simulink model "frdm_main"  (R2017a)
settings: Solver=FixedStepAuto  StartTime=0.0  StopTime=inf  RelTol=1e-3  EnableMultiTasking=on
libraries: frdmtfcshieldlib x5, frdmkl25zlib x2
settings Model: SimulationMode=external  ExtModeTrigDuration=5  Creator=WARA  LastModifiedBy=WARA
settings OptimizationCC: PassReuseOutputArgsThreshold=0  MaxStackSize=64
settings DebuggingCC: ParameterTunabilityLossMsg=error
settings HardwareCC: ProdBitPerPointer=32  ProdBitPerSizeT=32  ProdBitPerPtrDiffT=32  ProdLargestAtomicInteger=Long  ProdLargestAtomicFloat=Double  ProdWordSize=32  ProdHWDeviceType=ARM Compatible->ARM Cortex  UseEmbeddedCoderFeatures=off
settings SFSimCC: MATLABDynamicMemAlloc=off
settings RTWCC: SystemTargetFile=ert.tlc  HardwareBoard=NXP FRDM-KL25Z  TLCOptions=-aInlineSetEventsForThisBaseRateFcn=TLC_FALSE -aSuppressMultiTaskScheduler=TLC_FALSE -aRateBasedStepFcn=1  TemplateMakefile=ert_default_tmf  Description=Embedded Coder  GenerateReport=on  Toolchain=GNU Tools for ARM Embedded Processors  LaunchReport=on
settings CodeAppCC: ForceParamTrailComments=on  OperatorAnnotations=on  MATLABSourceComments=on
settings ERTTargetCC: ERTCustomFileBanners=off  SupportContinuousTime=on  SupportNonInlinedSFcns=on  RemoveResetFunc=off  ModelStepFunctionPrototypeControlCompliant=off

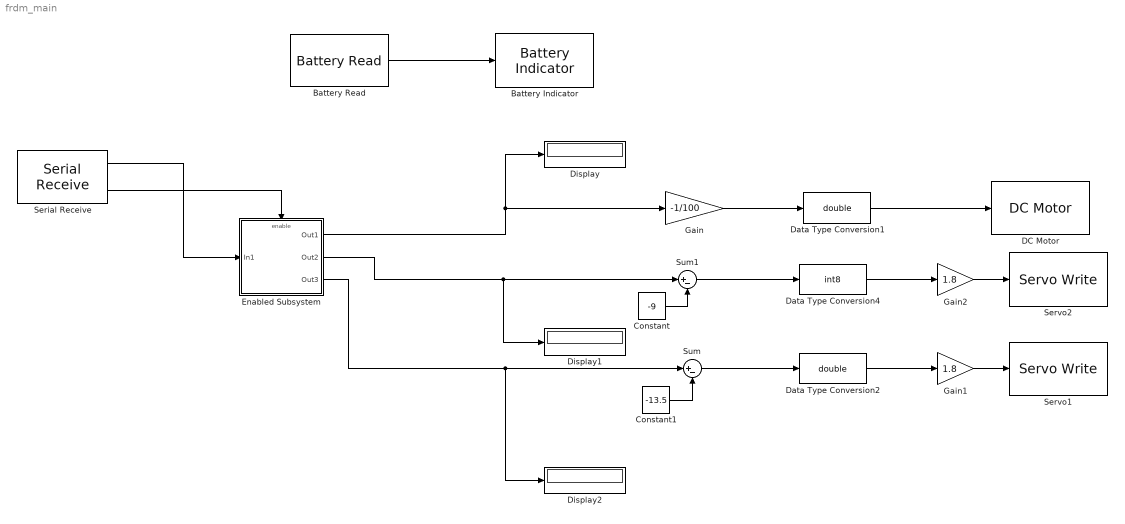
== system frdm_main ==
  Battery Indicator : frdmtfcshieldlib/Battery Indicator
      settings: SourceProductName=Simulink Coder Support Package for NXP FRDM-KL25Z Board  SourceProductBaseCode=EC_FREEDOM_BOARD
  Battery Read : frdmtfcshieldlib/Battery Read  SampleTime=0.1
      settings: SourceProductName=Simulink Coder Support Package for NXP FRDM-KL25Z Board  SourceProductBaseCode=EC_FREEDOM_BOARD
  Constant : Constant  Value=-9
  Constant1 : Constant  Value=-13.5
  DC Motor : frdmtfcshieldlib/DC Motor  WhichMotor=B
      settings: SourceProductName=Simulink Coder Support Package for NXP FRDM-KL25Z Board  SourceProductBaseCode=EC_FREEDOM_BOARD
  Data Type Conversion1 : DataTypeConversion  OutDataTypeStr=double
  Data Type Conversion2 : DataTypeConversion  OutDataTypeStr=double
  Data Type Conversion4 : DataTypeConversion  OutDataTypeStr=int8
  Display : Display
  Display1 : Display
  Display2 : Display
  Enabled Subsystem : Subsystem  TreatAsAtomicUnit=on
  Gain : Gain  Gain=-1/100
  Gain1 : Gain  Gain=1.8
  Gain2 : Gain  Gain=1.8
  Serial Receive : frdmkl25zlib/Serial Receive  uart=UART2  DataType=int8  DataLength=4  SampleTime=0.1
      settings: SourceProductName=Simulink Coder Support Package for NXP FRDM-KL25Z Board  SourceProductBaseCode=EC_FREEDOM_BOARD
  Servo1 : frdmtfcshieldlib/Servo Write  WhichServo=0  minAngle=-30  maxAngle=70
      settings: SourceProductName=Simulink Coder Support Package for NXP FRDM-KL25Z Board  SourceProductBaseCode=EC_FREEDOM_BOARD
  Servo2 : frdmtfcshieldlib/Servo Write  WhichServo=1  minAngle=-30  maxAngle=70
      settings: SourceProductName=Simulink Coder Support Package for NXP FRDM-KL25Z Board  SourceProductBaseCode=EC_FREEDOM_BOARD
  Sum : Sum  Inputs=|+-
  Sum1 : Sum  Inputs=|+-
  wires:
  Data Type Conversion1/1 -> DC Motor/1
  Enabled Subsystem/1(Out1) -> Display/1, Gain/1
  Sum1/1 -> Data Type Conversion4/1
  Gain/1 -> Data Type Conversion1/1
  Data Type Conversion4/1 -> Gain2/1
  Serial Receive/1 -> Enabled Subsystem/1(In1)
  Battery Read/1 -> Battery Indicator/1
  Data Type Conversion2/1 -> Gain1/1
  Gain2/1 -> Servo2/1
  Enabled Subsystem/3(Out3) -> Display2/1, Sum/1
  Constant1/1 -> Sum/2
  Constant/1 -> Sum1/2
  Gain1/1 -> Servo1/1
  Sum/1 -> Data Type Conversion2/1
  Serial Receive/2 -> Enabled Subsystem/Enable
  Enabled Subsystem/2(Out2) -> Display1/1, Sum1/1

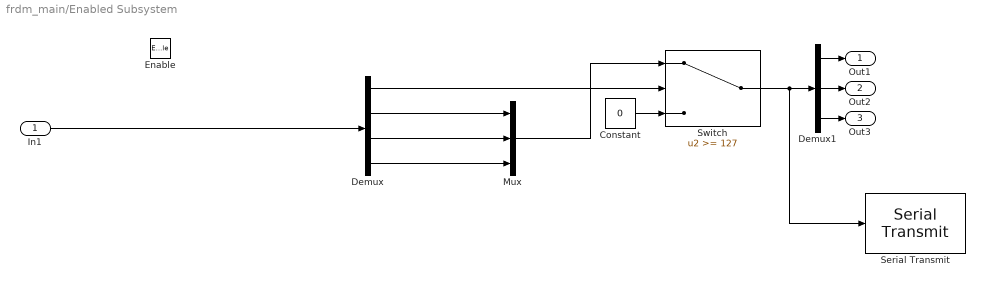
== system frdm_main/Enabled Subsystem ==
  In1 : Inport
  Enable : EnablePort
  Constant : Constant  Value=0
  Demux : Demux
  Demux1 : Demux  Outputs=3
  Mux : Mux  Inputs=3
  Serial Transmit : frdmkl25zlib/Serial Transmit  uart=UART2  sendmode=putc
      settings: SourceProductName=Simulink Coder Support Package for NXP FRDM-KL25Z Board  SourceProductBaseCode=EC_FREEDOM_BOARD
  Switch : Switch  Threshold=127
  Out1 : Outport
  Out2 : Outport  Port=2
  Out3 : Outport  Port=3
  wires:
  In1/1 -> Demux/1
  Demux/1 -> Switch/2
  Demux/2 -> Mux/1
  Demux/3 -> Mux/2
  Demux/4 -> Mux/3
  Mux/1 -> Switch/1
  Constant/1 -> Switch/3
  Switch/1 -> Serial Transmit/1, Demux1/1
  Demux1/1 -> Out1/1
  Demux1/2 -> Out2/1
  Demux1/3 -> Out3/1
